simulink model "chapter4"  (R2018a)
settings: Solver=VariableStepAuto  StartTime=0.0  StopTime=50  RelTol=1e-3
values from neighbouring files (symbols this model uses):
  C = [cs1       ,0        ,0        ,-cs1                   ,0              ,L1*cs1                       ,0 ... (first row only)    [vibs_project.m]
  K = [kt1+ks1,0       ,0       ,-ks1                  ,0                      ,L1*ks1                        ,0 ... (first row only)    [vibs_project.m]
  kt1 = 847000,kt2=2000000,kt3=2000000,ks1=300000,ks2=967430,ks3=155800,ks4=20000000    [vibs_project.m]
  M = [m1 ,0 ,0 ,0 ,0 ,0 ,0 ... (first row only)    [vibs_project.m]
  t1 = 0    [vibs_project.m]
  t2 = t1+(L1+L2)/V    [vibs_project.m]
  t3 = t2+(L5+L4+L3-L2)/V    [vibs_project.m]
undefined symbols (not defined in the file or in its folder): kt2, kt3
settings Model: Creator=Toshiba  LastModifiedBy=Toshiba

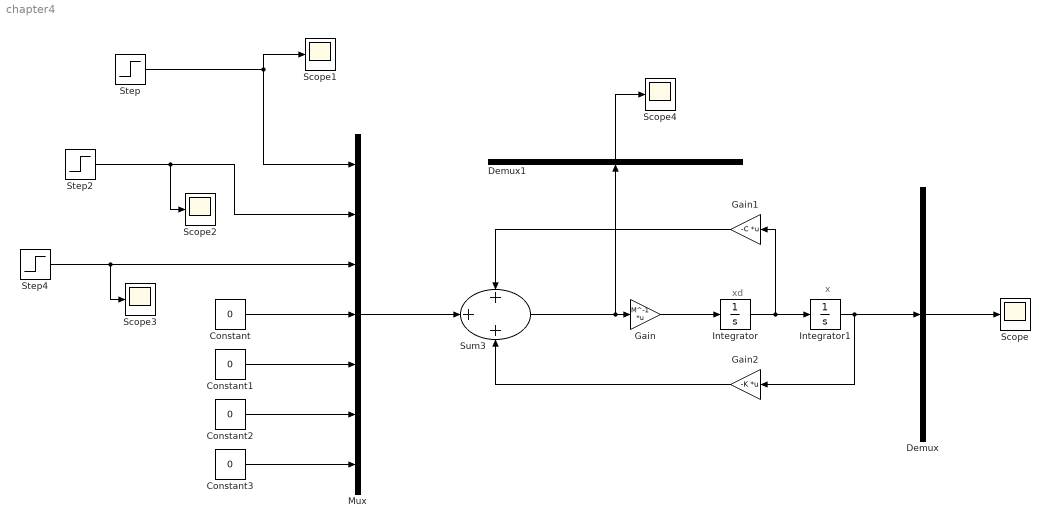
== system chapter4 ==
  note: x
  note: xd
  Constant{,1..3} (4 alike) : Constant  Value=0
  Demux : Demux  Outputs=7
  Demux1 : Demux  Outputs=7
  Gain : Gain  Gain=M^-1  Multiplication=Matrix(K*u)
  Gain1 : Gain  Gain=-C  Multiplication=Matrix(K*u)
  Gain2 : Gain  Gain=-K  Multiplication=Matrix(K*u)
  Integrator : Integrator
  Integrator1 : Integrator
  Mux : Mux  Inputs=7
  Scope{,1..4} (5 alike) : Scope
  Step : Step  Time=t1  After=kt1  SampleTime=0
  Step2 : Step  Time=t2  After=kt2  SampleTime=0
  Step4 : Step  Time=t3  After=kt3  SampleTime=0
  Sum3 : Sum  Inputs=+++
  wires:
  Step/1 -> Scope1/1, Mux/1
  Step2/1 -> Scope2/1, Mux/2
  Step4/1 -> Mux/3, Scope3/1
  Constant3/1 -> Mux/7
  Constant2/1 -> Mux/6
  Constant1/1 -> Mux/5
  Constant/1 -> Mux/4
  Mux/1 -> Sum3/2
  Sum3/1 -> Demux1/1, Gain/1
  Gain/1 -> Integrator/1
  Integrator/1 -> Gain1/1, Integrator1/1
  Gain2/1 -> Sum3/3
  Gain1/1 -> Sum3/1
  Integrator1/1 -> Gain2/1, Demux/1
  Demux/4 -> Scope/1
  Demux1/4 -> Scope4/1
